simulink model "Monitoring"  (R2020a)
settings: Solver=FixedStepDiscrete  StartTime=0.0  StopTime=inf  FixedStep=0.01  RelTol=1e-3  EnableMultiTasking=on
model workspace (MATLAB code in the model file):
  | clear
  | clc
  | 
  | PORT = 2324;
  | 
  | echotcpip('on', PORT)
  | tcp = tcpip('127.0.0.1',PORT);
  | fopen(tcp);
  | tcp.Status
  | sendString = "%.3f, %.3f, %.3f, %.3f, %.3f, %.3f, %.3f, %.3f, %.3f\n";
  | receiveString = "%f, %f, %f, %f, %f, %f, %f, %f, %f\n";
libraries: aerolibanimutils x1
settings Model: Creator=guilherme  LastModifiedBy=leona
settings SolverCC: AutoInsertRateTranBlk=on
settings DataIOCC: SaveOutput=off  SaveTime=off  ReturnWorkspaceOutputs=off
settings OptimizationCC: DefaultParameterBehavior=Inlined  InlineInvariantSignals=on  EnhancedBackFolding=on  PassReuseOutputArgsAs=Individual arguments  StateBitsets=on  DataBitsets=on  ZeroExternalMemoryAtStartup=off  ZeroInternalMemoryAtStartup=off  NoFixptDivByZeroProtection=on  LifeSpan=1  OptimizeBlockOrder=speed  DifferentSizesBufferReuse=on  EfficientTunableParamExpr=on
settings DebuggingCC: ParameterTunabilityLossMsg=error  ArithmeticOperatorsInVariantConditions=warning
settings HardwareCC: ProdBitPerPointer=32  ProdBitPerSizeT=32  ProdBitPerPtrDiffT=32  ProdLargestAtomicFloat=None  ProdIntDivRoundTo=Floor  ProdWordSize=32  ProdHWDeviceType=Generic->Custom
settings SFSimCC: SimUseLocalCustomCode=off  MATLABDynamicMemAlloc=off  CustomCodeUndefinedFunction=UseInterfaceOnly
settings RTWCC: SystemTargetFile=ert.tlc  TLCOptions=-p0  GenCodeOnly=on  TemplateMakefile=ert_default_tmf  GenerateReport=on  RTWVerbose=off  RTWUseLocalCustomCode=off  IncludeHyperlinkInReport=on  LaunchReport=on
settings CodeAppCC: ForceParamTrailComments=on  IgnoreCustomStorageClasses=off  OperatorAnnotations=on  SimulinkDataObjDesc=on  SFDataObjDesc=on  CustomSymbolStrGlobalVar=rt$N$M  CustomSymbolStrType=$N$M  CustomSymbolStrFcn=$N$M$F  CustomSymbolStrMacro=$N$M  InsertBlockDesc=on
settings ERTTargetCC: TargetLangStandard=C99 (ISO)  CodeReplacementLibrary=ISO_C  GenerateSampleERTMain=on  IncludeMdlTerminateFcn=off  SuppressErrorStatus=on  SupportAbsoluteTime=off  PurelyIntegerCode=on  SupportNonFinite=off  SupportComplex=off  InlinedParameterPlacement=NonHierarchical  RootIOFormat=Structure reference  ERTCustomFileTemplate=example_file_process.tlc

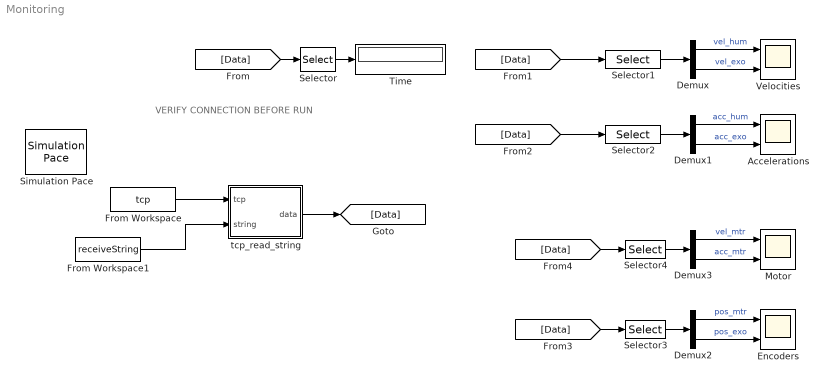
== system Monitoring ==
  note: VERIFY CONNECTION BEFORE RUN
  Accelerations : Scope  NumInputPorts=2
  Demux{,1..3} (4 alike) : Demux  Outputs=2
  Encoders : Scope  NumInputPorts=2
  From Workspace : FromWorkspace  VariableName=tcp
  From Workspace1 : FromWorkspace  VariableName=receiveString
  Motor : Scope  NumInputPorts=2
  Selector : Selector  InputPortWidth=9  IndexOptions=Index vector (dialog)  Indices=[1]  OutputSizes=1
  Selector1 : Selector  InputPortWidth=9  IndexOptions=Index vector (dialog)  Indices=[2 3]  OutputSizes=1
  Selector2 : Selector  InputPortWidth=9  IndexOptions=Index vector (dialog)  Indices=[4 5]  OutputSizes=1
  Selector3 : Selector  InputPortWidth=9  IndexOptions=Index vector (dialog)  Indices=[6 7]  OutputSizes=1
  Selector4 : Selector  InputPortWidth=9  IndexOptions=Index vector (dialog)  Indices=[8 9]  OutputSizes=1
  Simulation Pace : aerolibanimutils/Simulation Pace  SimulationPace=1  SleepMode=Auto  OutputPaceError=off  SampleTime=-1
  Time : Display
  Velocities : Scope  NumInputPorts=2
  tcp_read_string : MATLAB Function  TreatAsAtomicUnit=on
  wires:
  Selector/1 -> Time/1
  Demux/1 -> Velocities/1  "vel_hum"
  Demux/2 -> Velocities/2  "vel_exo"
  Selector1/1 -> Demux/1
  Selector2/1 -> Demux1/1
  Demux1/2 -> Accelerations/2  "acc_exo"
  Demux1/1 -> Accelerations/1  "acc_hum"
  Demux2/1 -> Encoders/1  "pos_mtr"
  Demux2/2 -> Encoders/2  "pos_exo"
  Selector3/1 -> Demux2/1
  [Data] -> Selector/1
  [Data] -> Selector1/1
  [Data] -> Selector2/1
  [Data] -> Selector3/1
  [Data] -> Selector4/1
  Selector4/1 -> Demux3/1
  Demux3/2 -> Motor/2  "acc_mtr"
  Demux3/1 -> Motor/1  "vel_mtr"
  tcp_read_string/1(data) -> [Data]
  From Workspace/1 -> tcp_read_string/1(tcp)
  From Workspace1/1 -> tcp_read_string/2(string)

== matlab function Monitoring/tcp_read_string ==
  data: tcp input; data output; string input
function data = fcn(tcp, string)
data = fscanf(tcp, string);
